simulink model "untitled1"  (R2024b)
settings: Solver=VariableStepAuto  StartTime=0.0  StopTime=10.0  RelTol=1e-3
values from neighbouring files (symbols this model uses):
  czasskok = 500    [MocGrzalkiPI.m]    (also in PrawyCz1.m = 0; PrawyCz2.m; Spr2.m = 1000; Sprb.m = 1000)
  dPg = 0.1*Pgn    (= 1000)    [PrawyCz2.m]    (also in labPI.m)
  k = 3.5 / 1000    (= 0.0035)    [MocGrzalkiPI.m]    (also in PrawyCz2.m; Sprb.m; gpt02.m; labPI.m)
  T = 760    [MocGrzalkiPI.m]    (also in PrawyCz2.m; Sprb.m = 1855; gpt02.m; labPI.m)
  Tw20 = 15    [MocGrzalkiPI.m]    (also in PrawyCz2.m; Sprb.m; gpt02.m; labPI.m)
  Tzero = 40    [MocGrzalkiPI.m]    (also in PrawyCz2.m = 60; gpt02.m; labPI.m)
settings Model: Creator=pawli  LastModifiedBy=pawli

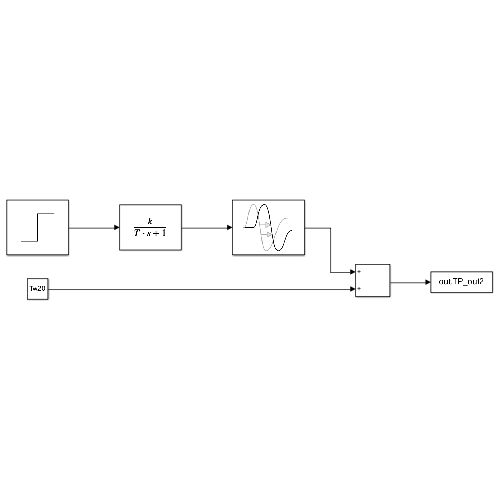
[thumbnail: Simulink's stored preview of the top-level diagram]
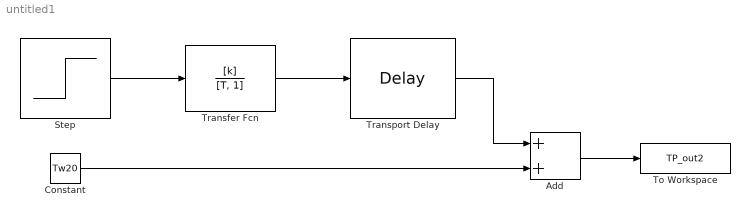
== system untitled1 ==
  Add : Sum
  Constant : Constant  Value=Tw20
  Step : Step  Time=0  After=dPg  SampleTime=0
  To Workspace : ToWorkspace  VariableName=TP_out2  SampleTime=-1
  Transfer Fcn : TransferFcn  Numerator=[k]  Denominator=[T, 1]
  Transport Delay : TransportDelay  DelayTime=Tzero+czasskok
  wires:
  Step/1 -> Transfer Fcn/1
  Transfer Fcn/1 -> Transport Delay/1
  Constant/1 -> Add/2
  Transport Delay/1 -> Add/1
  Add/1 -> To Workspace/1
